simulink model "bibli_SM_QUEVAL_20240121_R2021a"  (Simulink 9.3)
settings: Solver=VariableStepAuto  StartTime=0.0  StopTime=10  MaxStep=1e-3  RelTol=1e-3
values from neighbouring files (symbols this model uses):
  Fif = 0.259*3    (= 0.777)    [param_PMSM.m]
  J = 0.5    [param_EESM.m]    (also in param_EESMdampers.m; param_PMSM.m)
  Ld = 1.59e-2    (= 0.0159)    [param_EESM.m]    (also in param_EESMdampers.m; param_PMSM.m)
  Lq = 1.59e-2    (= 0.0159)    [param_EESM.m]    (also in param_EESMdampers.m; param_PMSM.m)
  npp = 2    [param_EESM.m]    (also in param_EESMdampers.m; param_PMSM.m)
undefined symbols (not defined in the file or in its folder): iao_pd_si, ibo_pd_si, ico_pd_si, Ts
undefined symbols (not defined in the file): Clark, fd, InvClark, INVL, M, R
libraries: powerlib x42
(part 2 of 2)

== system bibli_SM_QUEVAL_20240121_R2021a/MS bobiné/MS bobiné/Park1/Rotation ==
  cos : Inport
  sin : Inport  Port=2
  alpha : Inport  Port=3
  beta : Inport  Port=4
  Product{,1..3} (4 alike) : Product  InputSameDT=on  RndMeth=Zero  SaturateOnIntegerOverflow=on  OutDataTypeStr=Inherit: Same as first input
  Sum : Sum  InputSameDT=on  SaturateOnIntegerOverflow=on  OutDataTypeStr=Inherit: Same as first input
  Sum1 : Sum  Inputs=-+  InputSameDT=on  SaturateOnIntegerOverflow=on  OutDataTypeStr=Inherit: Same as first input
  d : Outport  InitialOutput=0  VectorParamsAs1DForOutWhenUnconnected=off
  q : Outport  Port=2  InitialOutput=0  VectorParamsAs1DForOutWhenUnconnected=off
  wires:
  alpha/1 -> Product2/1, Product/2
  beta/1 -> Product3/2, Product1/2
  Sum1/1 -> q/1
  Sum/1 -> d/1
  Product3/1 -> Sum1/2
  Product2/1 -> Sum1/1
  cos/1 -> Product3/1, Product/1
  sin/1 -> Product2/2, Product1/1
  Product1/1 -> Sum/2
  Product/1 -> Sum/1

== system bibli_SM_QUEVAL_20240121_R2021a/MS bobiné/MS bobiné/Parkinv1/ClarkInv ==
  alpha : Inport
  beta : Inport  Port=2
  o : Inport  Port=3
  "ClarkInv " : StateSpace  A=[]  B=[]  C=[]  D=K  InitialCondition=0  mask(Matrix Gain){K=InvClark}
      mask prompts: K "Gain matrix:"
      mask help: Matrix Gain.
      mask Help: Multiplies input vector by entered matrix to produce output vector (y=Au).
      mask Display: disp('K')
  Demux : Demux  Outputs=3
      settings: DisplayOption=none
  Mux : Mux  Inputs=3
  a : Outport  InitialOutput=0  VectorParamsAs1DForOutWhenUnconnected=off
  b : Outport  Port=2  InitialOutput=0  VectorParamsAs1DForOutWhenUnconnected=off
  c : Outport  Port=3  InitialOutput=0  VectorParamsAs1DForOutWhenUnconnected=off
  wires:
  Demux/3 -> c/1
  Demux/2 -> b/1
  Demux/1 -> a/1
  "ClarkInv "/1 -> Demux/1
  Mux/1 -> "ClarkInv "/1
  o/1 -> Mux/3
  beta/1 -> Mux/2
  alpha/1 -> Mux/1

== system bibli_SM_QUEVAL_20240121_R2021a/MS bobiné/MS bobiné/Parkinv1/Rotation Inverse ==
  cos : Inport
  sin : Inport  Port=2
  d : Inport  Port=3
  q : Inport  Port=4
  Product{,1..3} (4 alike) : Product  InputSameDT=on  RndMeth=Zero  SaturateOnIntegerOverflow=on  OutDataTypeStr=Inherit: Same as first input
  Sum : Sum  Inputs=+-  InputSameDT=on  SaturateOnIntegerOverflow=on  OutDataTypeStr=Inherit: Same as first input
  Sum1 : Sum  InputSameDT=on  SaturateOnIntegerOverflow=on  OutDataTypeStr=Inherit: Same as first input
  alpha : Outport  InitialOutput=0  VectorParamsAs1DForOutWhenUnconnected=off
  beta : Outport  Port=2  InitialOutput=0  VectorParamsAs1DForOutWhenUnconnected=off
  wires:
  d/1 -> Product2/1, Product/2
  q/1 -> Product3/2, Product1/2
  Sum1/1 -> beta/1
  Sum/1 -> alpha/1
  Product3/1 -> Sum1/2
  Product2/1 -> Sum1/1
  cos/1 -> Product3/1, Product/1
  sin/1 -> Product2/2, Product1/1
  Product1/1 -> Sum/2
  Product/1 -> Sum/1

== system bibli_SM_QUEVAL_20240121_R2021a/MS bobiné amortisseurs/MS bobiné amortisseurs/Park/Clark ==
  a : Inport
  b : Inport  Port=2
  c : Inport  Port=3
  "Clark " : StateSpace  A=[]  B=[]  C=[]  D=K  InitialCondition=0  mask(Matrix Gain){K=Clark}
      mask prompts: K "Gain matrix:"
      mask help: Matrix Gain.
      mask Help: Multiplies input vector by entered matrix to produce output vector (y=Au).
      mask Display: disp('K')
  Demux : Demux  Outputs=3
      settings: DisplayOption=none
  Mux : Mux  Inputs=3
  alpha : Outport  InitialOutput=0  VectorParamsAs1DForOutWhenUnconnected=off
  beta : Outport  Port=2  InitialOutput=0  VectorParamsAs1DForOutWhenUnconnected=off
  o : Outport  Port=3  InitialOutput=0  VectorParamsAs1DForOutWhenUnconnected=off
  wires:
  Demux/3 -> o/1
  Demux/2 -> beta/1
  Demux/1 -> alpha/1
  "Clark "/1 -> Demux/1
  Mux/1 -> "Clark "/1
  c/1 -> Mux/3
  b/1 -> Mux/2
  a/1 -> Mux/1

== system bibli_SM_QUEVAL_20240121_R2021a/MS bobiné amortisseurs/MS bobiné amortisseurs/Park/Rotation ==
  cos : Inport
  sin : Inport  Port=2
  alpha : Inport  Port=3
  beta : Inport  Port=4
  Product{,1..3} (4 alike) : Product  InputSameDT=on  RndMeth=Zero  SaturateOnIntegerOverflow=on  OutDataTypeStr=Inherit: Same as first input
  Sum : Sum  InputSameDT=on  SaturateOnIntegerOverflow=on  OutDataTypeStr=Inherit: Same as first input
  Sum1 : Sum  Inputs=-+  InputSameDT=on  SaturateOnIntegerOverflow=on  OutDataTypeStr=Inherit: Same as first input
  d : Outport  InitialOutput=0  VectorParamsAs1DForOutWhenUnconnected=off
  q : Outport  Port=2  InitialOutput=0  VectorParamsAs1DForOutWhenUnconnected=off
  wires:
  alpha/1 -> Product2/1, Product/2
  beta/1 -> Product3/2, Product1/2
  Sum1/1 -> q/1
  Sum/1 -> d/1
  Product3/1 -> Sum1/2
  Product2/1 -> Sum1/1
  cos/1 -> Product3/1, Product/1
  sin/1 -> Product2/2, Product1/1
  Product1/1 -> Sum/2
  Product/1 -> Sum/1

== system bibli_SM_QUEVAL_20240121_R2021a/MS bobiné amortisseurs/MS bobiné amortisseurs/Parkinv/ClarkInv ==
  alpha : Inport
  beta : Inport  Port=2
  o : Inport  Port=3
  "ClarkInv " : StateSpace  A=[]  B=[]  C=[]  D=K  InitialCondition=0  mask(Matrix Gain){K=InvClark}
      mask prompts: K "Gain matrix:"
      mask help: Matrix Gain.
      mask Help: Multiplies input vector by entered matrix to produce output vector (y=Au).
      mask Display: disp('K')
  Demux : Demux  Outputs=3
      settings: DisplayOption=none
  Mux : Mux  Inputs=3
  a : Outport  InitialOutput=0  VectorParamsAs1DForOutWhenUnconnected=off
  b : Outport  Port=2  InitialOutput=0  VectorParamsAs1DForOutWhenUnconnected=off
  c : Outport  Port=3  InitialOutput=0  VectorParamsAs1DForOutWhenUnconnected=off
  wires:
  Demux/3 -> c/1
  Demux/2 -> b/1
  Demux/1 -> a/1
  "ClarkInv "/1 -> Demux/1
  Mux/1 -> "ClarkInv "/1
  o/1 -> Mux/3
  beta/1 -> Mux/2
  alpha/1 -> Mux/1

== system bibli_SM_QUEVAL_20240121_R2021a/MS bobiné amortisseurs/MS bobiné amortisseurs/Parkinv/Rotation Inverse ==
  cos : Inport
  sin : Inport  Port=2
  d : Inport  Port=3
  q : Inport  Port=4
  Product{,1..3} (4 alike) : Product  InputSameDT=on  RndMeth=Zero  SaturateOnIntegerOverflow=on  OutDataTypeStr=Inherit: Same as first input
  Sum : Sum  Inputs=+-  InputSameDT=on  SaturateOnIntegerOverflow=on  OutDataTypeStr=Inherit: Same as first input
  Sum1 : Sum  InputSameDT=on  SaturateOnIntegerOverflow=on  OutDataTypeStr=Inherit: Same as first input
  alpha : Outport  InitialOutput=0  VectorParamsAs1DForOutWhenUnconnected=off
  beta : Outport  Port=2  InitialOutput=0  VectorParamsAs1DForOutWhenUnconnected=off
  wires:
  d/1 -> Product2/1, Product/2
  q/1 -> Product3/2, Product1/2
  Sum1/1 -> beta/1
  Sum/1 -> alpha/1
  Product3/1 -> Sum1/2
  Product2/1 -> Sum1/1
  cos/1 -> Product3/1, Product/1
  sin/1 -> Product2/2, Product1/1
  Product1/1 -> Sum/2
  Product/1 -> Sum/1

== system bibli_SM_QUEVAL_20240121_R2021a/PMSM/PMSM/Park/Clark ==
  a : Inport
  b : Inport  Port=2
  c : Inport  Port=3
  "Clark " : StateSpace  A=[]  B=[]  C=[]  D=K  InitialCondition=0  mask(Matrix Gain){K=Clark}
      mask prompts: K "Gain matrix:"
      mask help: Matrix Gain.
      mask Help: Multiplies input vector by entered matrix to produce output vector (y=Au).
      mask Display: disp('K')
  Demux : Demux  Outputs=3
      settings: DisplayOption=none
  Mux : Mux  Inputs=3
  alpha : Outport  InitialOutput=0  VectorParamsAs1DForOutWhenUnconnected=off
  beta : Outport  Port=2  InitialOutput=0  VectorParamsAs1DForOutWhenUnconnected=off
  o : Outport  Port=3  InitialOutput=0  VectorParamsAs1DForOutWhenUnconnected=off
  wires:
  Demux/3 -> o/1
  Demux/2 -> beta/1
  Demux/1 -> alpha/1
  "Clark "/1 -> Demux/1
  Mux/1 -> "Clark "/1
  c/1 -> Mux/3
  b/1 -> Mux/2
  a/1 -> Mux/1

== system bibli_SM_QUEVAL_20240121_R2021a/PMSM/PMSM/Park/Rotation ==
  cos : Inport
  sin : Inport  Port=2
  alpha : Inport  Port=3
  beta : Inport  Port=4
  Product{,1..3} (4 alike) : Product  InputSameDT=on  SaturateOnIntegerOverflow=on  OutDataTypeStr=Inherit: Same as first input
  Sum : Sum  InputSameDT=on  SaturateOnIntegerOverflow=on  OutDataTypeStr=Inherit: Same as first input
  Sum1 : Sum  Inputs=-+  InputSameDT=on  SaturateOnIntegerOverflow=on  OutDataTypeStr=Inherit: Same as first input
  d : Outport  InitialOutput=0  VectorParamsAs1DForOutWhenUnconnected=off
  q : Outport  Port=2  InitialOutput=0  VectorParamsAs1DForOutWhenUnconnected=off
  wires:
  alpha/1 -> Product2/1, Product/2
  beta/1 -> Product3/2, Product1/2
  Sum1/1 -> q/1
  Sum/1 -> d/1
  Product3/1 -> Sum1/2
  Product2/1 -> Sum1/1
  cos/1 -> Product3/1, Product/1
  sin/1 -> Product2/2, Product1/1
  Product1/1 -> Sum/2
  Product/1 -> Sum/1

== system bibli_SM_QUEVAL_20240121_R2021a/PMSM/PMSM/Parkinv/ClarkInv ==
  alpha : Inport
  beta : Inport  Port=2
  o : Inport  Port=3
  "ClarkInv " : StateSpace  A=[]  B=[]  C=[]  D=K  InitialCondition=0  mask(Matrix Gain){K=InvClark}
      mask prompts: K "Gain matrix:"
      mask help: Matrix Gain.
      mask Help: Multiplies input vector by entered matrix to produce output vector (y=Au).
      mask Display: disp('K')
  Demux : Demux  Outputs=3
      settings: DisplayOption=none
  Mux : Mux  Inputs=3
  a : Outport  InitialOutput=0  VectorParamsAs1DForOutWhenUnconnected=off
  b : Outport  Port=2  InitialOutput=0  VectorParamsAs1DForOutWhenUnconnected=off
  c : Outport  Port=3  InitialOutput=0  VectorParamsAs1DForOutWhenUnconnected=off
  wires:
  Demux/3 -> c/1
  Demux/2 -> b/1
  Demux/1 -> a/1
  "ClarkInv "/1 -> Demux/1
  Mux/1 -> "ClarkInv "/1
  o/1 -> Mux/3
  beta/1 -> Mux/2
  alpha/1 -> Mux/1

== system bibli_SM_QUEVAL_20240121_R2021a/PMSM/PMSM/Parkinv/Rotation Inverse ==
  cos : Inport
  sin : Inport  Port=2
  d : Inport  Port=3
  q : Inport  Port=4
  Product{,1..3} (4 alike) : Product  InputSameDT=on  SaturateOnIntegerOverflow=on  OutDataTypeStr=Inherit: Same as first input
  Sum : Sum  Inputs=+-  InputSameDT=on  SaturateOnIntegerOverflow=on  OutDataTypeStr=Inherit: Same as first input
  Sum1 : Sum  InputSameDT=on  SaturateOnIntegerOverflow=on  OutDataTypeStr=Inherit: Same as first input
  alpha : Outport  InitialOutput=0  VectorParamsAs1DForOutWhenUnconnected=off
  beta : Outport  Port=2  InitialOutput=0  VectorParamsAs1DForOutWhenUnconnected=off
  wires:
  d/1 -> Product2/1, Product/2
  q/1 -> Product3/2, Product1/2
  Sum1/1 -> beta/1
  Sum/1 -> alpha/1
  Product3/1 -> Sum1/2
  Product2/1 -> Sum1/1
  cos/1 -> Product3/1, Product/1
  sin/1 -> Product2/2, Product1/1
  Product1/1 -> Sum/2
  Product/1 -> Sum/1
